simulink model "QuadCentreClosedCoupling"  (R2022b)
settings: Solver=ode4  StartTime=0.0  StopTime=10  FixedStep=1e-3  RelTol=1e-3
undefined symbols (not defined in the file): t1, t2, Vus0
settings Model: Creator=Serious Chimp  LastModifiedBy=Serious Chimp
settings SolverCC: EnableFixedStepZeroCrossing=on
settings OptimizationCC: ReuseModelBlockBuffer=on

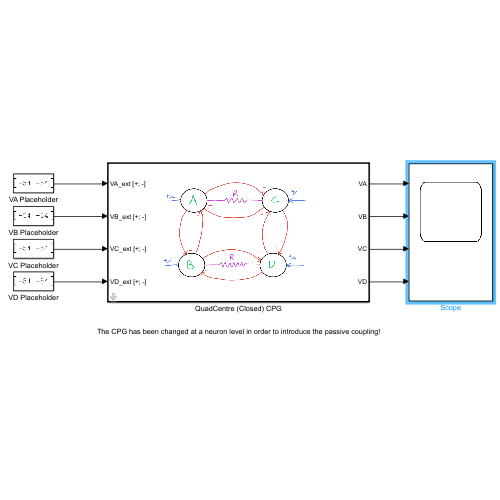
[thumbnail: Simulink's stored preview of the top-level diagram]
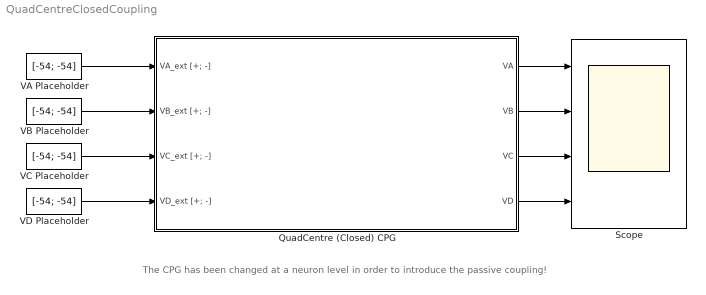
== system QuadCentreClosedCoupling ==
  note: The CPG has been changed at a neuron level in order to introduce the passive coupling!
  QuadCentre (Closed) CPG : Subsystem  TreatAsAtomicUnit=on  mask{tau_s_A=t1, tau_us_A=t2, gSyn_excitatory_A=0.5, gSyn_inhibitory_A=0.5, tauSyn_excitatory_A=50, tauSyn_inhibitory_A=50, GB_A=-40, tau_s_B=t1, tau_us_B=t2, gSyn_excitatory_B=0.5, gSyn_inhibitory_B=0.5, tauSyn_excitatory_B=50, tauSyn_inhibitory_B=50, GB_B=-35, tau_s_C=t1, tau_us_C=t2, gSyn_excitatory_C=0.5, gSyn_inhibitory_C=0.5, tauSyn_excitatory_C=50, tauSyn_inhibitory_C=50, GB_C=-35, tau_s_D=t1, tau_us_D=t2, gSyn_excitatory_D=0.5, gSyn_inhibitory_D=0.5, tauSyn_excitatory_D=50, tauSyn_inhibitory_D=50, GB_D=-40, GB_excitatory=-40, R=200}
      mask prompts: tau_s_A "A - tau_s"; tau_us_A "A - tau_us"; gSyn_excitatory_A "A - Excitatory Synaptic Conductance, gSyn_excitatory"; gSyn_inhibitory_A "A - Inhibitory Synaptic Conductance, gSyn_inhibitory"; tauSyn_excitatory_A "A - Excitatory Synaptic Time Constant, tauSyn_excitatory"; tauSyn_inhibitory_A "A - Inhibitory Synaptic Time Constant, tauSyn_inhibitory"; GB_A "A - Inhibitory Synapse Threshold, GB_A"; tau_s_B "B - tau_s"; tau_us_B "B - tau_us"; gSyn_excitatory_B "B - Excitatory Synaptic Conductance, gSyn_excitatory"; gSyn_inhibitory_B "B - Inhibitory Synaptic Conductance, gSyn_inhibitory"; tauSyn_excitatory_B "B - Excitatory Synaptic Time Constant, tauSyn_excitatory"; tauSyn_inhibitory_B "B - Inhibitory Synaptic Time Constant, tauSyn_inhibitory"; GB_B "B - Inhibitory Synapse Threshold, GB_B"; tau_s_C "C - tau_s"; tau_us_C "C - tau_us"; gSyn_excitatory_C "C - Excitatory Synaptic Conductance, gSyn_excitatory"; gSyn_inhibitory_C "C - Inhibitory Synaptic Conductance, gSyn_inhibitory"; tauSyn_excitatory_C "C - Excitatory Synaptic Time Constant, tauSyn_excitatory"; tauSyn_inhibitory_C "C - Inhibitory Synaptic Time Constant, tauSyn_inhibitory"; GB_C "C - Inhibitory Synapse Threshold, GB_C"; tau_s_D "D - tau_s"; tau_us_D "D - tau_us"; gSyn_excitatory_D "D - Excitatory Synaptic Conductance, gSyn_excitatory"; gSyn_inhibitory_D "D - Inhibitory Synaptic Conductance, gSyn_inhibitory"; tauSyn_excitatory_D "D - Excitatory Synaptic Time Constant, tauSyn_excitatory"; tauSyn_inhibitory_D "D - Inhibitory Synaptic Time Constant, tauSyn_inhibitory"; GB_D "D - Inhibitory Synapse Threshold, GB_D"; GB_excitatory "Excitatory Synapse Gate Threshold, GB_excitatory"; R "Coupling Resistance, R"
      mask Display: image('$imagefile'); % Use "Edit Image" on toolstrip to change.
  Scope : Scope  NumInputPorts=4
  VA Placeholder : Constant  Value=[-54; -54]
  VB Placeholder : Constant  Value=[-54; -54]
  VC Placeholder : Constant  Value=[-54; -54]
  VD Placeholder : Constant  Value=[-54; -54]
  wires:
  QuadCentre (Closed) CPG/1(VA) -> Scope/1
  QuadCentre (Closed) CPG/2(VB) -> Scope/2
  QuadCentre (Closed) CPG/3(VC) -> Scope/3
  QuadCentre (Closed) CPG/4(VD) -> Scope/4
  VA Placeholder/1 -> QuadCentre (Closed) CPG/1(VA_ext [+; -])
  VB Placeholder/1 -> QuadCentre (Closed) CPG/2(VB_ext [+; -])
  VD Placeholder/1 -> QuadCentre (Closed) CPG/4(VD_ext [+; -])
  VC Placeholder/1 -> QuadCentre (Closed) CPG/3(VC_ext [+; -])

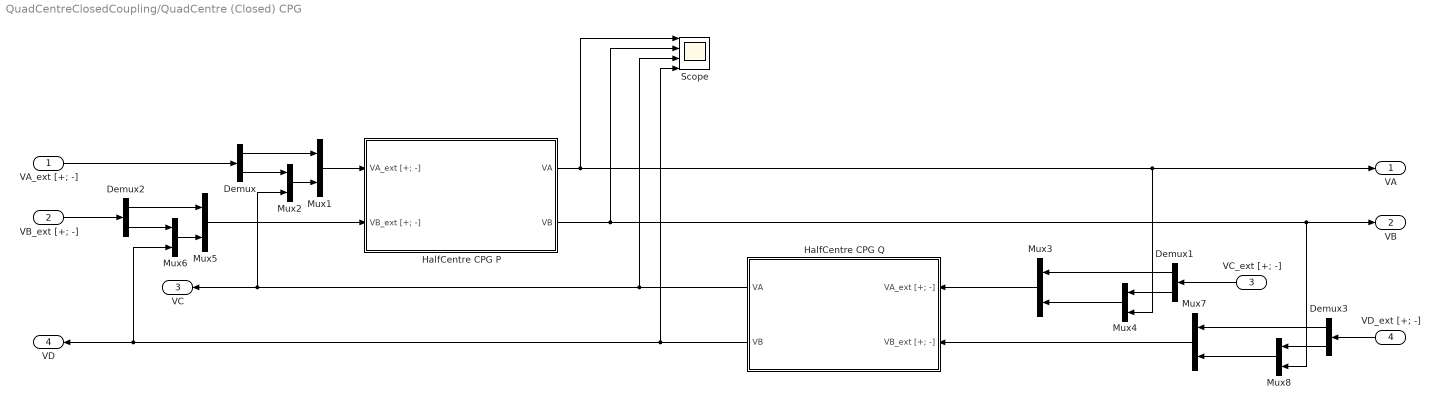
== system QuadCentreClosedCoupling/QuadCentre (Closed) CPG ==
  VA_ext [+; -] : Inport
  VB_ext [+; -] : Inport  Port=2
  VC_ext [+; -] : Inport  Port=3
  VD_ext [+; -] : Inport  Port=4
  Demux{,1..3} (4 alike) : Demux  Outputs=2
  HalfCentre CPG P : Subsystem  TreatAsAtomicUnit=on  mask{tau_s_A=t1, tau_us_A=t2, gSyn_excitatory_A=gSyn_excitatory_A, gSyn_inhibitory_A=gSyn_inhibitory_A, tauSyn_excitatory_A=tauSyn_excitatory_A, tauSyn_inhibitory_A=tauSyn_inhibitory_A, GB_A=GB_A, tau_s_B=t1, tau_us_B=t2, gSyn_excitatory_B=gSyn_excitatory_B, gSyn_inhibitory_B=gSyn_inhibitory_B, tauSyn_excitatory_B=tauSyn_excitatory_B, tauSyn_inhibitory_B=tauSyn_inhibitory_B, GB_B=GB_B, GB_excitatory=GB_excitatory}
      mask prompts: tau_s_A "A - tau_s"; tau_us_A "A - tau_us"; gSyn_excitatory_A "A - Excitatory Synaptic Conductance, gSyn_excitatory"; gSyn_inhibitory_A "A - Inhibitory Synaptic Conductance, gSyn_inhibitory"; tauSyn_excitatory_A "A - Excitatory Synaptic Time Constant, tauSyn_excitatory"; tauSyn_inhibitory_A "A - Inhibitory Synaptic Time Constant, tauSyn_inhibitory"; GB_A "A - Inhibitory Synapse Threshold, GB_A"; tau_s_B "B - tau_s"; tau_us_B "B - tau_us"; gSyn_excitatory_B "B - Excitatory Synaptic Conductance, gSyn_excitatory"; gSyn_inhibitory_B "B - Inhibitory Synaptic Conductance, gSyn_inhibitory"; tauSyn_excitatory_B "B - Excitatory Synaptic Time Constant, tauSyn_excitatory"; tauSyn_inhibitory_B "B - Inhibitory Synaptic Time Constant, tauSyn_inhibitory"; GB_B "B - Inhibitory Synapse Threshold, GB_B"; GB_excitatory "Excitatory Gate Biases, GB_excitatory"
      mask Display: image('$imagefile'); % Use "Edit Image" on toolstrip to change.
  HalfCentre CPG Q : Subsystem  TreatAsAtomicUnit=on  mask{tau_s_A=t1, tau_us_A=t2, gSyn_excitatory_A=gSyn_excitatory_C, gSyn_inhibitory_A=gSyn_inhibitory_C, tauSyn_excitatory_A=tauSyn_excitatory_C, tauSyn_inhibitory_A=tauSyn_inhibitory_C, GB_A=GB_C, tau_s_B=t1, tau_us_B=t2, gSyn_excitatory_B=gSyn_excitatory_D, gSyn_inhibitory_B=gSyn_inhibitory_D, tauSyn_excitatory_B=tauSyn_excitatory_D, tauSyn_inhibitory_B=tauSyn_inhibitory_D, GB_B=GB_D, GB_excitatory=GB_excitatory}
      mask prompts: tau_s_A "A - tau_s"; tau_us_A "A - tau_us"; gSyn_excitatory_A "A - Excitatory Synaptic Conductance, gSyn_excitatory"; gSyn_inhibitory_A "A - Inhibitory Synaptic Conductance, gSyn_inhibitory"; tauSyn_excitatory_A "A - Excitatory Synaptic Time Constant, tauSyn_excitatory"; tauSyn_inhibitory_A "A - Inhibitory Synaptic Time Constant, tauSyn_inhibitory"; GB_A "A - Inhibitory Synapse Threshold, GB_A"; tau_s_B "B - tau_s"; tau_us_B "B - tau_us"; gSyn_excitatory_B "B - Excitatory Synaptic Conductance, gSyn_excitatory"; gSyn_inhibitory_B "B - Inhibitory Synaptic Conductance, gSyn_inhibitory"; tauSyn_excitatory_B "B - Excitatory Synaptic Time Constant, tauSyn_excitatory"; tauSyn_inhibitory_B "B - Inhibitory Synaptic Time Constant, tauSyn_inhibitory"; GB_B "B - Inhibitory Synapse Threshold, GB_B"; GB_excitatory "Excitatory Gate Biases, GB_excitatory"
      mask Display: image('$imagefile'); % Use "Edit Image" on toolstrip to change.
  Mux{1..8} (8 alike) : Mux  Inputs=2
  Scope : Scope  NumInputPorts=4
  VA : Outport
  VB : Outport  Port=2
  VC : Outport  Port=3
  VD : Outport  Port=4
  wires:
  Demux3/2 -> Mux8/1
  HalfCentre CPG P/2(VB) -> Mux8/2, VB/1, Scope/2
  Demux1/2 -> Mux4/1
  Demux3/1 -> Mux7/1
  Mux8/1 -> Mux7/2
  VD_ext [+; -]/1 -> Demux3/1
  Mux1/1 -> HalfCentre CPG P/1(VA_ext [+; -])
  Mux3/1 -> HalfCentre CPG Q/1(VA_ext [+; -])
  Demux/1 -> Mux1/1
  Demux2/1 -> Mux5/1
  Demux2/2 -> Mux6/1
  VC_ext [+; -]/1 -> Demux1/1
  Mux2/1 -> Mux1/2
  VB_ext [+; -]/1 -> Demux2/1
  Mux6/1 -> Mux5/2
  VA_ext [+; -]/1 -> Demux/1
  HalfCentre CPG P/1(VA) -> Scope/1, Mux4/2, VA/1
  Demux/2 -> Mux2/1
  Mux7/1 -> HalfCentre CPG Q/2(VB_ext [+; -])
  Mux5/1 -> HalfCentre CPG P/2(VB_ext [+; -])
  Mux4/1 -> Mux3/2
  Demux1/1 -> Mux3/1
  HalfCentre CPG Q/1(VA) -> Scope/3, Mux2/2, VC/1
  HalfCentre CPG Q/2(VB) -> Mux6/2, VD/1, Scope/4

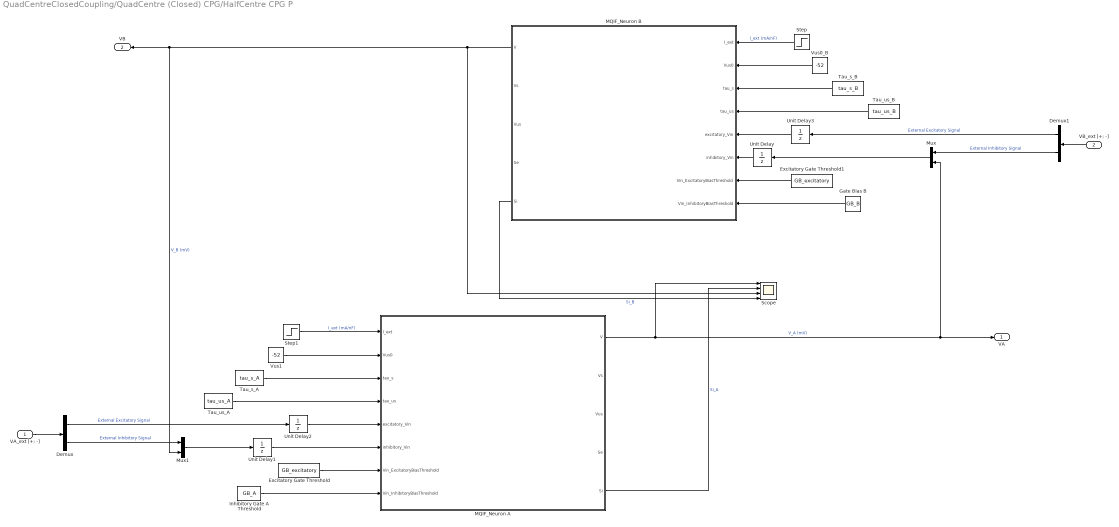
== system QuadCentreClosedCoupling/QuadCentre (Closed) CPG/HalfCentre CPG P ==
  VA_ext [+; -] : Inport
  VB_ext [+; -] : Inport  Port=2
  Demux : Demux  Outputs=2
  Demux1 : Demux  Outputs=2
  Excitatory Gate Threshold : Constant  Value=GB_excitatory
  Excitatory Gate Threshold1 : Constant  Value=GB_excitatory
  Gate BIas B : Constant  Value=GB_B
  Inhibitory Gate A Threshold : Constant  Value=GB_A
  MQIF_Neuron A : Subsystem  TreatAsAtomicUnit=on  mask{V0=-52, Vs0=-50, V_threshold=20, V_reset=-45, Vs_reset=7.5, delta_Vus=1.7, g_f=1.0, g_s=0.5, g_us=0.015, C=0.82, Ve_syn=0, Vi_syn=-90, g_syn_excitatory=gSyn_excitatory_A, g_syn_inhibitory=gSyn_inhibitory_A, tauSyn_excitatory=tauSyn_excitatory_A, tauSyn_inhibitory=tauSyn_inhibitory_A, k=250}
      mask prompts: V0 "Equilibrium V0"; Vs0 "Equilibrium Vs0"; V_threshold "Threshold for Spike, V_thresh"; V_reset "After-spike Reset Votlage, V_r"; Vs_reset "After-spike Reset Vs, Vs_r"; delta_Vus "Vus After-spike Memory, delta_Vus"; g_f "I Conductance, g_f"; g_s "I_us Conductance, g_s"; g_us "I_us Conductance, g_us"; C "Capacitance, C"; Ve_syn "Equilibrium Inhibitory Synapse Voltage, Ve_syn"; Vi_syn "Equilibrium Inhibitory Synapse Voltage, Vi_syn"; g_syn_excitatory "Excitatory Synapse Conductance, g_syn_excitatory"; g_syn_inhibitory "Inhibitory Synapse Conductance, g_syn_inhibitory"; tauSyn_excitatory "Excitatory Synapse Time Constant, tauSyn_excitatory"; tauSyn_inhibitory "Inhibitory Synapse Time Constant, tauSyn_inhibitory"; k "Speed/Rate Constant, k"
      mask DialogControl NeuronStateVariables Prompt: Parameters
  MQIF_Neuron B : Subsystem  TreatAsAtomicUnit=on  mask{V0=-52, Vs0=-50, V_threshold=20, V_reset=-45, Vs_reset=7.5, delta_Vus=1.7, g_f=1.0, g_s=0.5, g_us=0.015, C=0.82, Ve_syn=0, Vi_syn=-90, g_syn_excitatory=gSyn_excitatory_B, g_syn_inhibitory=gSyn_inhibitory_B, tauSyn_excitatory=tauSyn_excitatory_B, tauSyn_inhibitory=tauSyn_inhibitory_B, k=250}
      mask prompts: V0 "Equilibrium V0"; Vs0 "Equilibrium Vs0"; V_threshold "Threshold for Spike, V_thresh"; V_reset "After-spike Reset Votlage, V_r"; Vs_reset "After-spike Reset Vs, Vs_r"; delta_Vus "Vus After-spike Memory, delta_Vus"; g_f "I Conductance, g_f"; g_s "I_us Conductance, g_s"; g_us "I_us Conductance, g_us"; C "Capacitance, C"; Ve_syn "Equilibrium Inhibitory Synapse Voltage, Ve_syn"; Vi_syn "Equilibrium Inhibitory Synapse Voltage, Vi_syn"; g_syn_excitatory "Excitatory Synapse Conductance, g_syn_excitatory"; g_syn_inhibitory "Inhibitory Synapse Conductance, g_syn_inhibitory"; tauSyn_excitatory "Excitatory Synapse Time Constant, tauSyn_excitatory"; tauSyn_inhibitory "Inhibitory Synapse Time Constant, tauSyn_inhibitory"; k "Speed/Rate Constant, k"
      mask DialogControl NeuronStateVariables Prompt: Parameters
  Mux : Mux  Inputs=2
  Mux1 : Mux  Inputs=2
  Scope : Scope  NumInputPorts=4
  Step : Step  After=5  SampleTime=0
  Step1 : Step  After=5  SampleTime=0
  Tau_s_A : Constant  Value=tau_s_A
  Tau_s_B : Constant  Value=tau_s_B
  Tau_us_A : Constant  Value=tau_us_A
  Tau_us_B : Constant  Value=tau_us_B
  Unit Delay : UnitDelay  InitialCondition=[-54; -54]  SampleTime=-1  HasFrameUpgradeWarning=on
  Unit Delay1 : UnitDelay  InitialCondition=[-54; -54]  SampleTime=-1  HasFrameUpgradeWarning=on
  Unit Delay2 : UnitDelay  InitialCondition=-54  SampleTime=-1  HasFrameUpgradeWarning=on
  Unit Delay3 : UnitDelay  InitialCondition=-54  SampleTime=-1  HasFrameUpgradeWarning=on
  Vus0_B : Constant  Value=-52
  Vus1 : Constant  Value=-52
  VA : Outport
  VB : Outport  Port=2
  wires:
  Vus0_B/1 -> MQIF_Neuron B/2(Vus0)
  Unit Delay/1 -> MQIF_Neuron B/6(inhibitory_Vin)
  Inhibitory Gate A Threshold/1 -> MQIF_Neuron A/8(Vin_InhibitoryBiasThreshold)
  Tau_us_B/1 -> MQIF_Neuron B/4(tau_us)
  Vus1/1 -> MQIF_Neuron A/2(Vus0)
  Step1/1 -> MQIF_Neuron A/1(I_ext)  "I_ext (mA/nF)"
  Tau_s_A/1 -> MQIF_Neuron A/3(tau_s)
  Tau_s_B/1 -> MQIF_Neuron B/3(tau_s)
  Tau_us_A/1 -> MQIF_Neuron A/4(tau_us)
  Step/1 -> MQIF_Neuron B/1(I_ext)  "I_ext (mA/nF)"
  Unit Delay1/1 -> MQIF_Neuron A/6(inhibitory_Vin)
  Gate BIas B/1 -> MQIF_Neuron B/8(Vin_InhibitoryBiasThreshold)
  VB_ext [+; -]/1 -> Demux1/1
  Mux/1 -> Unit Delay/1
  Mux1/1 -> Unit Delay1/1
  VA_ext [+; -]/1 -> Demux/1
  Excitatory Gate Threshold/1 -> MQIF_Neuron A/7(Vin_ExcitatoryBiasThreshold)
  Demux/1 -> Unit Delay2/1  "External Excitatory Signal"
  MQIF_Neuron A/1(V) -> Scope/1, VA/1, Mux/2  "V_A (mV)"
  Unit Delay3/1 -> MQIF_Neuron B/5(excitatory_Vin)
  Demux/2 -> Mux1/1  "External Inhibitory Signal"
  Unit Delay2/1 -> MQIF_Neuron A/5(excitatory_Vin)
  Demux1/2 -> Mux/1  "External Inhibitory Signal"
  Demux1/1 -> Unit Delay3/1  "External Excitatory Signal"
  Excitatory Gate Threshold1/1 -> MQIF_Neuron B/7(Vin_ExcitatoryBiasThreshold)
  MQIF_Neuron B/1(V) -> Scope/3, VB/1, Mux1/2  "V_B (mV)"
  MQIF_Neuron A/5(Si) -> Scope/2  "Si_A"
  MQIF_Neuron B/5(Si) -> Scope/4  "Si_B"

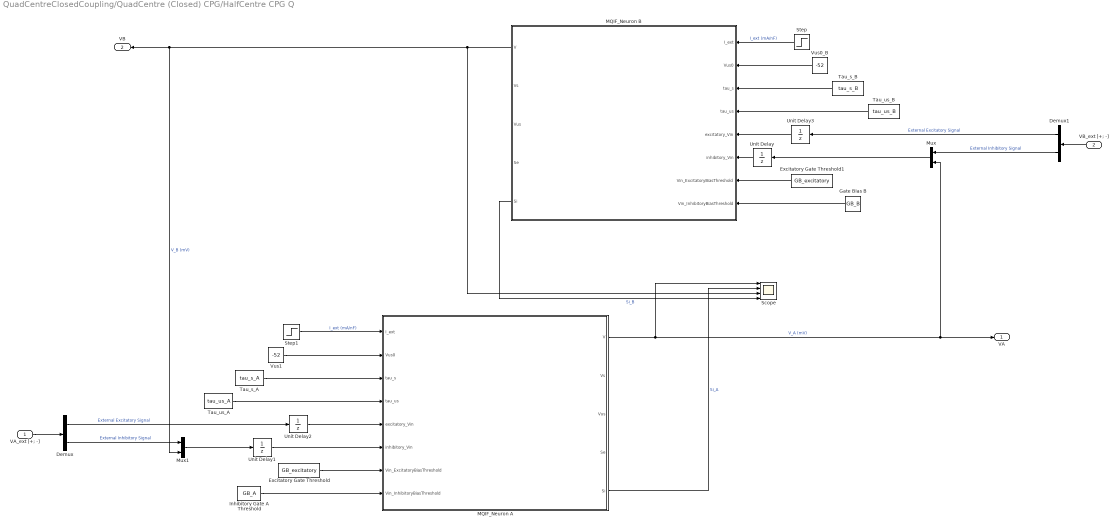
== system QuadCentreClosedCoupling/QuadCentre (Closed) CPG/HalfCentre CPG Q ==
  VA_ext [+; -] : Inport
  VB_ext [+; -] : Inport  Port=2
  Demux : Demux  Outputs=2
  Demux1 : Demux  Outputs=2
  Excitatory Gate Threshold : Constant  Value=GB_excitatory
  Excitatory Gate Threshold1 : Constant  Value=GB_excitatory
  Gate BIas B : Constant  Value=GB_B
  Inhibitory Gate A Threshold : Constant  Value=GB_A
  MQIF_Neuron A : Subsystem  TreatAsAtomicUnit=on  mask{V0=-52, Vs0=-50, V_threshold=20, V_reset=-45, Vs_reset=7.5, delta_Vus=1.7, g_f=1.0, g_s=0.5, g_us=0.015, C=0.82, Ve_syn=0, Vi_syn=-90, g_syn_excitatory=gSyn_excitatory_C, g_syn_inhibitory=gSyn_inhibitory_C, tauSyn_excitatory=tauSyn_excitatory_C, tauSyn_inhibitory=tauSyn_inhibitory_C, k=250}
      mask prompts: V0 "Equilibrium V0"; Vs0 "Equilibrium Vs0"; V_threshold "Threshold for Spike, V_thresh"; V_reset "After-spike Reset Votlage, V_r"; Vs_reset "After-spike Reset Vs, Vs_r"; delta_Vus "Vus After-spike Memory, delta_Vus"; g_f "I Conductance, g_f"; g_s "I_us Conductance, g_s"; g_us "I_us Conductance, g_us"; C "Capacitance, C"; Ve_syn "Equilibrium Inhibitory Synapse Voltage, Ve_syn"; Vi_syn "Equilibrium Inhibitory Synapse Voltage, Vi_syn"; g_syn_excitatory "Excitatory Synapse Conductance, g_syn_excitatory"; g_syn_inhibitory "Inhibitory Synapse Conductance, g_syn_inhibitory"; tauSyn_excitatory "Excitatory Synapse Time Constant, tauSyn_excitatory"; tauSyn_inhibitory "Inhibitory Synapse Time Constant, tauSyn_inhibitory"; k "Speed/Rate Constant, k"
      mask DialogControl NeuronStateVariables Prompt: Parameters
  MQIF_Neuron B : Subsystem  TreatAsAtomicUnit=on  mask{V0=-52, Vs0=-50, V_threshold=20, V_reset=-45, Vs_reset=7.5, delta_Vus=1.7, g_f=1.0, g_s=0.5, g_us=0.015, C=0.82, Ve_syn=0, Vi_syn=-90, g_syn_excitatory=gSyn_excitatory_D, g_syn_inhibitory=gSyn_inhibitory_D, tauSyn_excitatory=tauSyn_excitatory_D, tauSyn_inhibitory=tauSyn_inhibitory_D, k=250}
      mask prompts: V0 "Equilibrium V0"; Vs0 "Equilibrium Vs0"; V_threshold "Threshold for Spike, V_thresh"; V_reset "After-spike Reset Votlage, V_r"; Vs_reset "After-spike Reset Vs, Vs_r"; delta_Vus "Vus After-spike Memory, delta_Vus"; g_f "I Conductance, g_f"; g_s "I_us Conductance, g_s"; g_us "I_us Conductance, g_us"; C "Capacitance, C"; Ve_syn "Equilibrium Inhibitory Synapse Voltage, Ve_syn"; Vi_syn "Equilibrium Inhibitory Synapse Voltage, Vi_syn"; g_syn_excitatory "Excitatory Synapse Conductance, g_syn_excitatory"; g_syn_inhibitory "Inhibitory Synapse Conductance, g_syn_inhibitory"; tauSyn_excitatory "Excitatory Synapse Time Constant, tauSyn_excitatory"; tauSyn_inhibitory "Inhibitory Synapse Time Constant, tauSyn_inhibitory"; k "Speed/Rate Constant, k"
      mask DialogControl NeuronStateVariables Prompt: Parameters
  Mux : Mux  Inputs=2
  Mux1 : Mux  Inputs=2
  Scope : Scope  NumInputPorts=4
  Step : Step  After=5  SampleTime=0
  Step1 : Step  After=5  SampleTime=0
  Tau_s_A : Constant  Value=tau_s_A
  Tau_s_B : Constant  Value=tau_s_B
  Tau_us_A : Constant  Value=tau_us_A
  Tau_us_B : Constant  Value=tau_us_B
  Unit Delay : UnitDelay  InitialCondition=[-54; -54]  SampleTime=-1  HasFrameUpgradeWarning=on
  Unit Delay1 : UnitDelay  InitialCondition=[-54; -54]  SampleTime=-1  HasFrameUpgradeWarning=on
  Unit Delay2 : UnitDelay  InitialCondition=-54  SampleTime=-1  HasFrameUpgradeWarning=on
  Unit Delay3 : UnitDelay  InitialCondition=-54  SampleTime=-1  HasFrameUpgradeWarning=on
  Vus0_B : Constant  Value=-52
  Vus1 : Constant  Value=-52
  VA : Outport
  VB : Outport  Port=2
  wires:
  Vus0_B/1 -> MQIF_Neuron B/2(Vus0)
  Unit Delay/1 -> MQIF_Neuron B/6(inhibitory_Vin)
  Inhibitory Gate A Threshold/1 -> MQIF_Neuron A/8(Vin_InhibitoryBiasThreshold)
  Tau_us_B/1 -> MQIF_Neuron B/4(tau_us)
  Vus1/1 -> MQIF_Neuron A/2(Vus0)
  Step1/1 -> MQIF_Neuron A/1(I_ext)  "I_ext (mA/nF)"
  Tau_s_A/1 -> MQIF_Neuron A/3(tau_s)
  Tau_s_B/1 -> MQIF_Neuron B/3(tau_s)
  Tau_us_A/1 -> MQIF_Neuron A/4(tau_us)
  Step/1 -> MQIF_Neuron B/1(I_ext)  "I_ext (mA/nF)"
  Unit Delay1/1 -> MQIF_Neuron A/6(inhibitory_Vin)
  Gate BIas B/1 -> MQIF_Neuron B/8(Vin_InhibitoryBiasThreshold)
  VB_ext [+; -]/1 -> Demux1/1
  Mux/1 -> Unit Delay/1
  Mux1/1 -> Unit Delay1/1
  VA_ext [+; -]/1 -> Demux/1
  Excitatory Gate Threshold/1 -> MQIF_Neuron A/7(Vin_ExcitatoryBiasThreshold)
  Demux/1 -> Unit Delay2/1  "External Excitatory Signal"
  MQIF_Neuron A/1(V) -> Scope/1, VA/1, Mux/2  "V_A (mV)"
  Unit Delay3/1 -> MQIF_Neuron B/5(excitatory_Vin)
  Demux/2 -> Mux1/1  "External Inhibitory Signal"
  Unit Delay2/1 -> MQIF_Neuron A/5(excitatory_Vin)
  Demux1/2 -> Mux/1  "External Inhibitory Signal"
  Demux1/1 -> Unit Delay3/1  "External Excitatory Signal"
  Excitatory Gate Threshold1/1 -> MQIF_Neuron B/7(Vin_ExcitatoryBiasThreshold)
  MQIF_Neuron B/1(V) -> Scope/3, VB/1, Mux1/2  "V_B (mV)"
  MQIF_Neuron A/5(Si) -> Scope/2  "Si_A"
  MQIF_Neuron B/5(Si) -> Scope/4  "Si_B"

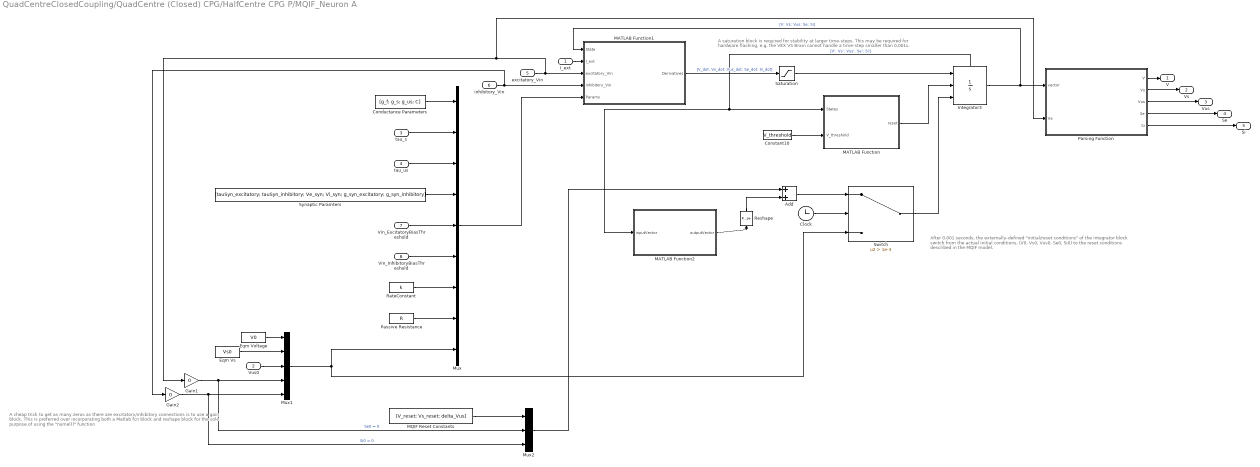
== system QuadCentreClosedCoupling/QuadCentre (Closed) CPG/HalfCentre CPG P/MQIF_Neuron A ==
  note: A saturation block is required for stability at larger time-steps. This may be required for hardware flashing, e.g. the VEX V5 Brain cannot handle a time-step smaller than 0.001s.
  note: After 0.001 seconds, the externally-defined "initial/reset conditions" of the integrator block switch from the actual initial conditions, (V0, Vs0, Vus0, Se0, Si0) to the reset conditions described in the MQIF model.
  note: A cheap trick to get as many zeros as there are excitatory/inhibitory connections
      | is to use a gain block. This is preferred over incorporating both a Matlab fcn block and reshape block for the sole purpose of using the "numel()" function
  I_ext : Inport
  Vus0 : Inport  Port=2
  tau_s : Inport  Port=3
  tau_us : Inport  Port=4
  excitatory_Vin : Inport  Port=5
  inhibitory_Vin : Inport  Port=6
  Vin_ExcitatoryBiasThreshold : Inport  Port=7
  Vin_InhibitoryBiasThreshold : Inport  Port=8
  Add : Sum
  Clock : Clock
  Conductance Parameters : Constant  Value=[g_f; g_s; g_us; C]
  Constant10 : Constant  Value=V_threshold
  Eqm Voltage : Constant  Value=V0
  Eqm Vs : Constant  Value=Vs0
  Gain1 : Gain  Gain=0
  Gain2 : Gain  Gain=0
  Integrator3 : Integrator  ExternalReset=rising  InitialConditionSource=external  InitialCondition=[V0 Vs0 Vus0]  ShowStatePort=on
  MATLAB Function : MATLAB Function  TreatAsAtomicUnit=on
  MATLAB Function1 : MATLAB Function  TreatAsAtomicUnit=on
  MATLAB Function2 : MATLAB Function  TreatAsAtomicUnit=on
  MQIF Reset Constants : Constant  Value=[V_reset; Vs_reset; delta_Vus]
  Mux : Mux  Inputs=9
  Mux1 : Mux  Inputs=5
  Mux2 : Mux  Inputs=3
  Parsing Function : MATLAB Function  TreatAsAtomicUnit=on
  Passive Resistance : Constant  Value=R
  RateConstant : Constant  Value=k
  Reshape : Reshape
  Saturation : Saturate  UpperLimit=1e4  LowerLimit=-1e4  LinearizeAsGain=off  ZeroCross=off
  Switch : Switch  Criteria=u2 > Threshold  Threshold=1e-3  SaturateOnIntegerOverflow=off  InputSameDT=off
  Synaptic Paramters : Constant  Value=[tauSyn_excitatory; tauSyn_inhibitory; Ve_syn; Vi_syn; g_syn_excitatory; g_syn_inhibitory]
  V : Outport
  Vs : Outport  Port=2
  Vus : Outport  Port=3
  Se : Outport  Port=4
  Si : Outport  Port=5
  wires:
  I_ext/1 -> MATLAB Function1/2(I_ext)
  Eqm Voltage/1 -> Mux1/1
  Vus0/1 -> Mux1/3
  Conductance Parameters/1 -> Mux/1
  tau_s/1 -> Mux/2
  tau_us/1 -> Mux/3
  Synaptic Paramters/1 -> Mux/4
  Mux/1 -> MATLAB Function1/5(Params)
  Constant10/1 -> MATLAB Function/2(V_threshold)
  Integrator3/1 -> MATLAB Function1/1(State), Parsing Function/1(vector)  "[V; Vs; Vus; Se; Si]"
  MATLAB Function/1(reset) -> Integrator3/2
  Clock/1 -> Switch/2
  MQIF Reset Constants/1 -> Mux2/1
  Switch/1 -> Integrator3/3
  MATLAB Function2/1(outputVector) -> Reshape/1
  MATLAB Function1/1(Derivatives) -> Saturation/1  "[V_dot; Vs_dot; Vus_dot; Se_dot; Si_dot]"
  Add/1 -> Switch/1
  Eqm Vs/1 -> Mux1/2
  inhibitory_Vin/1 -> Gain2/1, MATLAB Function1/4(inhibitory_Vin)
  Integrator3/State -> MATLAB Function2/1(inputVector), MATLAB Function/1(States)  "[V'; Vs'; Vus'; Se'; Si']"
  Vin_ExcitatoryBiasThreshold/1 -> Mux/5
  Saturation/1 -> Integrator3/1
  excitatory_Vin/1 -> Parsing Function/2(Ve), Gain1/1, MATLAB Function1/3(excitatory_Vin)
  RateConstant/1 -> Mux/7
  Mux1/1 -> Mux/9, Switch/3
  Vin_InhibitoryBiasThreshold/1 -> Mux/6
  Gain1/1 -> Mux1/4, Mux2/2  "Se0 = 0"
  Gain2/1 -> Mux2/3, Mux1/5  "Si0 = 0"
  Mux2/1 -> Add/1
  Reshape/1 -> Add/2
  Parsing Function/3(Vus) -> Vus/1
  Parsing Function/2(Vs) -> Vs/1
  Parsing Function/1(V) -> V/1
  Parsing Function/5(Si) -> Si/1
  Parsing Function/4(Se) -> Se/1
  Passive Resistance/1 -> Mux/8

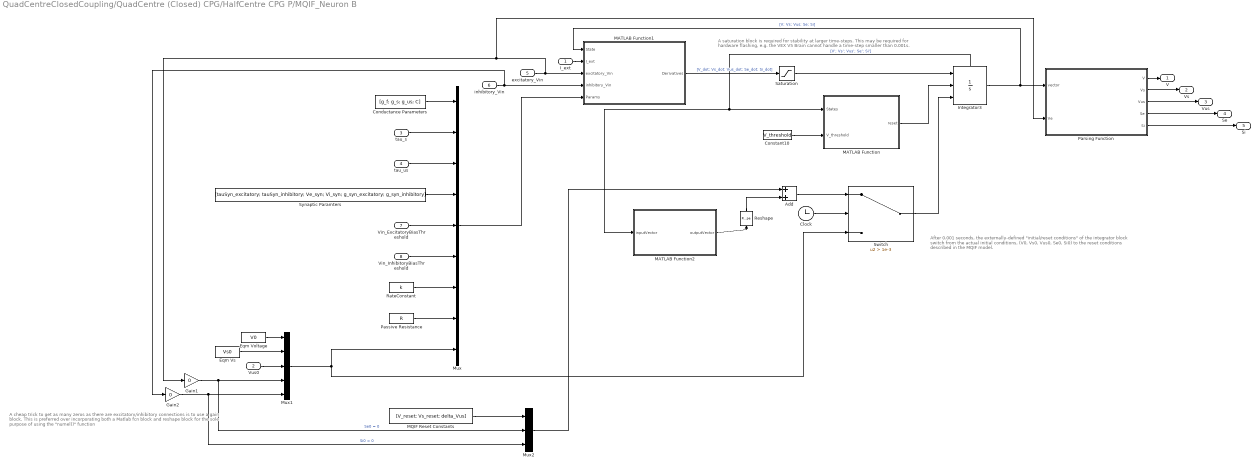
== system QuadCentreClosedCoupling/QuadCentre (Closed) CPG/HalfCentre CPG P/MQIF_Neuron B ==
  note: A saturation block is required for stability at larger time-steps. This may be required for hardware flashing, e.g. the VEX V5 Brain cannot handle a time-step smaller than 0.001s.
  note: After 0.001 seconds, the externally-defined "initial/reset conditions" of the integrator block switch from the actual initial conditions, (V0, Vs0, Vus0, Se0, Si0) to the reset conditions described in the MQIF model.
  note: A cheap trick to get as many zeros as there are excitatory/inhibitory connections
      | is to use a gain block. This is preferred over incorporating both a Matlab fcn block and reshape block for the sole purpose of using the "numel()" function
  I_ext : Inport
  Vus0 : Inport  Port=2
  tau_s : Inport  Port=3
  tau_us : Inport  Port=4
  excitatory_Vin : Inport  Port=5
  inhibitory_Vin : Inport  Port=6
  Vin_ExcitatoryBiasThreshold : Inport  Port=7
  Vin_InhibitoryBiasThreshold : Inport  Port=8
  Add : Sum
  Clock : Clock
  Conductance Parameters : Constant  Value=[g_f; g_s; g_us; C]
  Constant10 : Constant  Value=V_threshold
  Eqm Voltage : Constant  Value=V0
  Eqm Vs : Constant  Value=Vs0
  Gain1 : Gain  Gain=0
  Gain2 : Gain  Gain=0
  Integrator3 : Integrator  ExternalReset=rising  InitialConditionSource=external  InitialCondition=[V0 Vs0 Vus0]  ShowStatePort=on
  MATLAB Function : MATLAB Function  TreatAsAtomicUnit=on
  MATLAB Function1 : MATLAB Function  TreatAsAtomicUnit=on
  MATLAB Function2 : MATLAB Function  TreatAsAtomicUnit=on
  MQIF Reset Constants : Constant  Value=[V_reset; Vs_reset; delta_Vus]
  Mux : Mux  Inputs=9
  Mux1 : Mux  Inputs=5
  Mux2 : Mux  Inputs=3
  Parsing Function : MATLAB Function  TreatAsAtomicUnit=on
  Passive Resistance : Constant  Value=R
  RateConstant : Constant  Value=k
  Reshape : Reshape
  Saturation : Saturate  UpperLimit=1e4  LowerLimit=-1e4  LinearizeAsGain=off  ZeroCross=off
  Switch : Switch  Criteria=u2 > Threshold  Threshold=1e-3  SaturateOnIntegerOverflow=off  InputSameDT=off
  Synaptic Paramters : Constant  Value=[tauSyn_excitatory; tauSyn_inhibitory; Ve_syn; Vi_syn; g_syn_excitatory; g_syn_inhibitory]
  V : Outport
  Vs : Outport  Port=2
  Vus : Outport  Port=3
  Se : Outport  Port=4
  Si : Outport  Port=5
  wires:
  I_ext/1 -> MATLAB Function1/2(I_ext)
  Eqm Voltage/1 -> Mux1/1
  Vus0/1 -> Mux1/3
  Conductance Parameters/1 -> Mux/1
  tau_s/1 -> Mux/2
  tau_us/1 -> Mux/3
  Synaptic Paramters/1 -> Mux/4
  Mux/1 -> MATLAB Function1/5(Params)
  Constant10/1 -> MATLAB Function/2(V_threshold)
  Integrator3/1 -> MATLAB Function1/1(State), Parsing Function/1(vector)  "[V; Vs; Vus; Se; Si]"
  MATLAB Function/1(reset) -> Integrator3/2
  Clock/1 -> Switch/2
  MQIF Reset Constants/1 -> Mux2/1
  Switch/1 -> Integrator3/3
  MATLAB Function2/1(outputVector) -> Reshape/1
  MATLAB Function1/1(Derivatives) -> Saturation/1  "[V_dot; Vs_dot; Vus_dot; Se_dot; Si_dot]"
  Add/1 -> Switch/1
  Eqm Vs/1 -> Mux1/2
  inhibitory_Vin/1 -> Gain2/1, MATLAB Function1/4(inhibitory_Vin)
  Integrator3/State -> MATLAB Function2/1(inputVector), MATLAB Function/1(States)  "[V'; Vs'; Vus'; Se'; Si']"
  Vin_ExcitatoryBiasThreshold/1 -> Mux/5
  Saturation/1 -> Integrator3/1
  excitatory_Vin/1 -> Parsing Function/2(Ve), Gain1/1, MATLAB Function1/3(excitatory_Vin)
  RateConstant/1 -> Mux/7
  Mux1/1 -> Mux/9, Switch/3
  Vin_InhibitoryBiasThreshold/1 -> Mux/6
  Gain1/1 -> Mux1/4, Mux2/2  "Se0 = 0"
  Gain2/1 -> Mux2/3, Mux1/5  "Si0 = 0"
  Mux2/1 -> Add/1
  Reshape/1 -> Add/2
  Parsing Function/3(Vus) -> Vus/1
  Parsing Function/2(Vs) -> Vs/1
  Parsing Function/1(V) -> V/1
  Parsing Function/5(Si) -> Si/1
  Parsing Function/4(Se) -> Se/1
  Passive Resistance/1 -> Mux/8

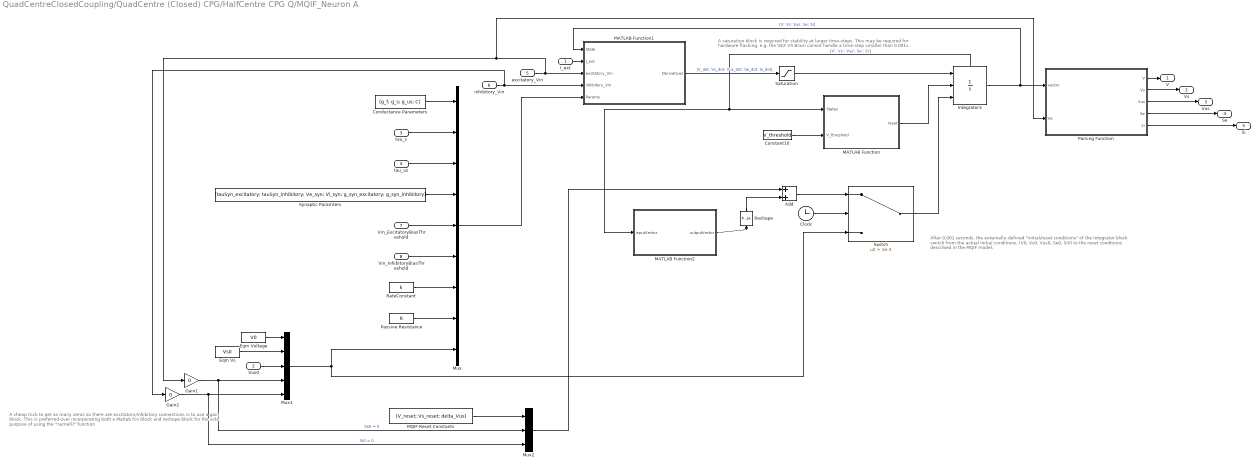
== system QuadCentreClosedCoupling/QuadCentre (Closed) CPG/HalfCentre CPG Q/MQIF_Neuron A ==
  note: A saturation block is required for stability at larger time-steps. This may be required for hardware flashing, e.g. the VEX V5 Brain cannot handle a time-step smaller than 0.001s.
  note: After 0.001 seconds, the externally-defined "initial/reset conditions" of the integrator block switch from the actual initial conditions, (V0, Vs0, Vus0, Se0, Si0) to the reset conditions described in the MQIF model.
  note: A cheap trick to get as many zeros as there are excitatory/inhibitory connections
      | is to use a gain block. This is preferred over incorporating both a Matlab fcn block and reshape block for the sole purpose of using the "numel()" function
  I_ext : Inport
  Vus0 : Inport  Port=2
  tau_s : Inport  Port=3
  tau_us : Inport  Port=4
  excitatory_Vin : Inport  Port=5
  inhibitory_Vin : Inport  Port=6
  Vin_ExcitatoryBiasThreshold : Inport  Port=7
  Vin_InhibitoryBiasThreshold : Inport  Port=8
  Add : Sum
  Clock : Clock
  Conductance Parameters : Constant  Value=[g_f; g_s; g_us; C]
  Constant10 : Constant  Value=V_threshold
  Eqm Voltage : Constant  Value=V0
  Eqm Vs : Constant  Value=Vs0
  Gain1 : Gain  Gain=0
  Gain2 : Gain  Gain=0
  Integrator3 : Integrator  ExternalReset=rising  InitialConditionSource=external  InitialCondition=[V0 Vs0 Vus0]  ShowStatePort=on
  MATLAB Function : MATLAB Function  TreatAsAtomicUnit=on
  MATLAB Function1 : MATLAB Function  TreatAsAtomicUnit=on
  MATLAB Function2 : MATLAB Function  TreatAsAtomicUnit=on
  MQIF Reset Constants : Constant  Value=[V_reset; Vs_reset; delta_Vus]
  Mux : Mux  Inputs=9
  Mux1 : Mux  Inputs=5
  Mux2 : Mux  Inputs=3
  Parsing Function : MATLAB Function  TreatAsAtomicUnit=on
  Passive Resistance : Constant  Value=R
  RateConstant : Constant  Value=k
  Reshape : Reshape
  Saturation : Saturate  UpperLimit=1e4  LowerLimit=-1e4  LinearizeAsGain=off  ZeroCross=off
  Switch : Switch  Criteria=u2 > Threshold  Threshold=1e-3  SaturateOnIntegerOverflow=off  InputSameDT=off
  Synaptic Paramters : Constant  Value=[tauSyn_excitatory; tauSyn_inhibitory; Ve_syn; Vi_syn; g_syn_excitatory; g_syn_inhibitory]
  V : Outport
  Vs : Outport  Port=2
  Vus : Outport  Port=3
  Se : Outport  Port=4
  Si : Outport  Port=5
  wires:
  I_ext/1 -> MATLAB Function1/2(I_ext)
  Eqm Voltage/1 -> Mux1/1
  Vus0/1 -> Mux1/3
  Conductance Parameters/1 -> Mux/1
  tau_s/1 -> Mux/2
  tau_us/1 -> Mux/3
  Synaptic Paramters/1 -> Mux/4
  Mux/1 -> MATLAB Function1/5(Params)
  Constant10/1 -> MATLAB Function/2(V_threshold)
  Integrator3/1 -> MATLAB Function1/1(State), Parsing Function/1(vector)  "[V; Vs; Vus; Se; Si]"
  MATLAB Function/1(reset) -> Integrator3/2
  Clock/1 -> Switch/2
  MQIF Reset Constants/1 -> Mux2/1
  Switch/1 -> Integrator3/3
  MATLAB Function2/1(outputVector) -> Reshape/1
  MATLAB Function1/1(Derivatives) -> Saturation/1  "[V_dot; Vs_dot; Vus_dot; Se_dot; Si_dot]"
  Add/1 -> Switch/1
  Eqm Vs/1 -> Mux1/2
  inhibitory_Vin/1 -> Gain2/1, MATLAB Function1/4(inhibitory_Vin)
  Integrator3/State -> MATLAB Function2/1(inputVector), MATLAB Function/1(States)  "[V'; Vs'; Vus'; Se'; Si']"
  Vin_ExcitatoryBiasThreshold/1 -> Mux/5
  Saturation/1 -> Integrator3/1
  excitatory_Vin/1 -> Parsing Function/2(Ve), Gain1/1, MATLAB Function1/3(excitatory_Vin)
  RateConstant/1 -> Mux/7
  Mux1/1 -> Mux/9, Switch/3
  Vin_InhibitoryBiasThreshold/1 -> Mux/6
  Gain1/1 -> Mux1/4, Mux2/2  "Se0 = 0"
  Gain2/1 -> Mux2/3, Mux1/5  "Si0 = 0"
  Mux2/1 -> Add/1
  Reshape/1 -> Add/2
  Parsing Function/3(Vus) -> Vus/1
  Parsing Function/2(Vs) -> Vs/1
  Parsing Function/1(V) -> V/1
  Parsing Function/5(Si) -> Si/1
  Parsing Function/4(Se) -> Se/1
  Passive Resistance/1 -> Mux/8

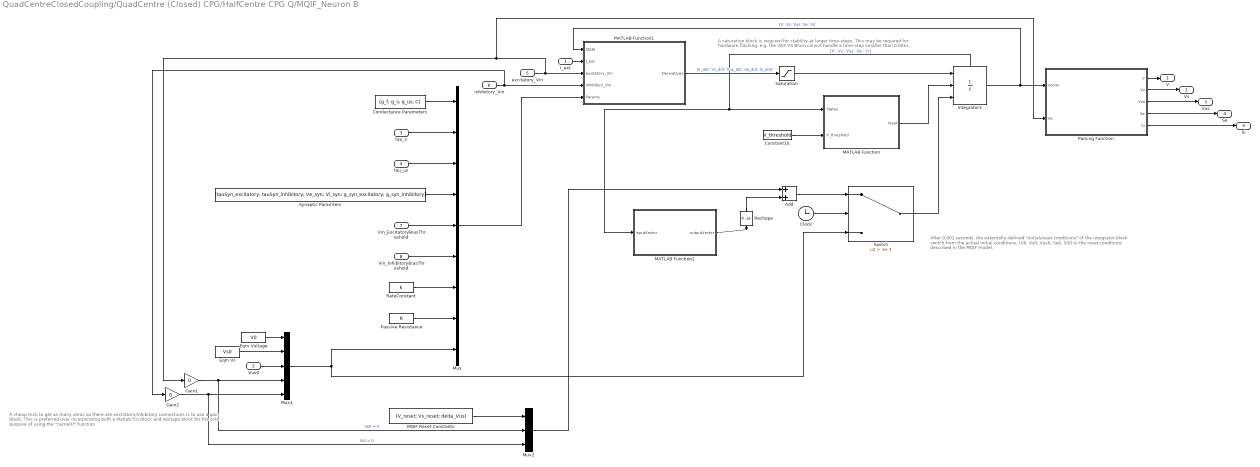
== system QuadCentreClosedCoupling/QuadCentre (Closed) CPG/HalfCentre CPG Q/MQIF_Neuron B ==
  note: A saturation block is required for stability at larger time-steps. This may be required for hardware flashing, e.g. the VEX V5 Brain cannot handle a time-step smaller than 0.001s.
  note: After 0.001 seconds, the externally-defined "initial/reset conditions" of the integrator block switch from the actual initial conditions, (V0, Vs0, Vus0, Se0, Si0) to the reset conditions described in the MQIF model.
  note: A cheap trick to get as many zeros as there are excitatory/inhibitory connections
      | is to use a gain block. This is preferred over incorporating both a Matlab fcn block and reshape block for the sole purpose of using the "numel()" function
  I_ext : Inport
  Vus0 : Inport  Port=2
  tau_s : Inport  Port=3
  tau_us : Inport  Port=4
  excitatory_Vin : Inport  Port=5
  inhibitory_Vin : Inport  Port=6
  Vin_ExcitatoryBiasThreshold : Inport  Port=7
  Vin_InhibitoryBiasThreshold : Inport  Port=8
  Add : Sum
  Clock : Clock
  Conductance Parameters : Constant  Value=[g_f; g_s; g_us; C]
  Constant10 : Constant  Value=V_threshold
  Eqm Voltage : Constant  Value=V0
  Eqm Vs : Constant  Value=Vs0
  Gain1 : Gain  Gain=0
  Gain2 : Gain  Gain=0
  Integrator3 : Integrator  ExternalReset=rising  InitialConditionSource=external  InitialCondition=[V0 Vs0 Vus0]  ShowStatePort=on
  MATLAB Function : MATLAB Function  TreatAsAtomicUnit=on
  MATLAB Function1 : MATLAB Function  TreatAsAtomicUnit=on
  MATLAB Function2 : MATLAB Function  TreatAsAtomicUnit=on
  MQIF Reset Constants : Constant  Value=[V_reset; Vs_reset; delta_Vus]
  Mux : Mux  Inputs=9
  Mux1 : Mux  Inputs=5
  Mux2 : Mux  Inputs=3
  Parsing Function : MATLAB Function  TreatAsAtomicUnit=on
  Passive Resistance : Constant  Value=R
  RateConstant : Constant  Value=k
  Reshape : Reshape
  Saturation : Saturate  UpperLimit=1e4  LowerLimit=-1e4  LinearizeAsGain=off  ZeroCross=off
  Switch : Switch  Criteria=u2 > Threshold  Threshold=1e-3  SaturateOnIntegerOverflow=off  InputSameDT=off
  Synaptic Paramters : Constant  Value=[tauSyn_excitatory; tauSyn_inhibitory; Ve_syn; Vi_syn; g_syn_excitatory; g_syn_inhibitory]
  V : Outport
  Vs : Outport  Port=2
  Vus : Outport  Port=3
  Se : Outport  Port=4
  Si : Outport  Port=5
  wires:
  I_ext/1 -> MATLAB Function1/2(I_ext)
  Eqm Voltage/1 -> Mux1/1
  Vus0/1 -> Mux1/3
  Conductance Parameters/1 -> Mux/1
  tau_s/1 -> Mux/2
  tau_us/1 -> Mux/3
  Synaptic Paramters/1 -> Mux/4
  Mux/1 -> MATLAB Function1/5(Params)
  Constant10/1 -> MATLAB Function/2(V_threshold)
  Integrator3/1 -> MATLAB Function1/1(State), Parsing Function/1(vector)  "[V; Vs; Vus; Se; Si]"
  MATLAB Function/1(reset) -> Integrator3/2
  Clock/1 -> Switch/2
  MQIF Reset Constants/1 -> Mux2/1
  Switch/1 -> Integrator3/3
  MATLAB Function2/1(outputVector) -> Reshape/1
  MATLAB Function1/1(Derivatives) -> Saturation/1  "[V_dot; Vs_dot; Vus_dot; Se_dot; Si_dot]"
  Add/1 -> Switch/1
  Eqm Vs/1 -> Mux1/2
  inhibitory_Vin/1 -> Gain2/1, MATLAB Function1/4(inhibitory_Vin)
  Integrator3/State -> MATLAB Function2/1(inputVector), MATLAB Function/1(States)  "[V'; Vs'; Vus'; Se'; Si']"
  Vin_ExcitatoryBiasThreshold/1 -> Mux/5
  Saturation/1 -> Integrator3/1
  excitatory_Vin/1 -> Parsing Function/2(Ve), Gain1/1, MATLAB Function1/3(excitatory_Vin)
  RateConstant/1 -> Mux/7
  Mux1/1 -> Mux/9, Switch/3
  Vin_InhibitoryBiasThreshold/1 -> Mux/6
  Gain1/1 -> Mux1/4, Mux2/2  "Se0 = 0"
  Gain2/1 -> Mux2/3, Mux1/5  "Si0 = 0"
  Mux2/1 -> Add/1
  Reshape/1 -> Add/2
  Parsing Function/3(Vus) -> Vus/1
  Parsing Function/2(Vs) -> Vs/1
  Parsing Function/1(V) -> V/1
  Parsing Function/5(Si) -> Si/1
  Parsing Function/4(Se) -> Se/1
  Passive Resistance/1 -> Mux/8

== matlab function QuadCentreClosedCoupling/QuadCentre (Closed) CPG/HalfCentre CPG Q/MQIF_Neuron B/MATLAB Function2 ==
  data: inputVector input; outputVector output
% This function is required to make sure that the MQIF neuron is input
% agnostic, (can handle any number of excitatory/inhibitory connections).
% 
% We require a matrix that can extract Vus (scalar), Se and Si (vectors of
% arbitrary length), and ignore the other values. This is because these
% values are "remembered" after each action potential and are required in
% the subsequent resetting of states.

function outputVector = generalisedMatrix(inputVector)
    % Get the size of the input vector
    n = length(inputVector);

    % Create a square matrix of zeros
    Matrix = zeros(n);

    % Set the (3, 3) element to 1
    Matrix(3, 3) = 1;

    % Set the values for every row i, starting from the fourth row
    for i = 4:n
        Matrix(i, i) = 1;
    end

    outputVector = Matrix*inputVector;
end

== matlab function QuadCentreClosedCoupling/QuadCentre (Closed) CPG/HalfCentre CPG Q/MQIF_Neuron B/Parsing Function ==
  data: vector input; V output; Vs output; Vus output; Ve input; Se output; Si output
% This fcn parses through the vectorised input signal, to output the
% various states through the enclosing mask's outports. It is designed to
% be input agnostic, (i.e. the neuron can handle any number of excitatory/inhibitory
% connections, and it outputs Se and Si as vectorised signals).

function [V,Vs,Vus,Se,Si] = InputAgnosticDemux(vector, Ve)
    V = vector(1);
    Vs = vector(2);
    Vus = vector(3);
    Se = vector(4:numel(Ve)+3);
    Si = vector(numel(Ve)+4:end);
end

== matlab function QuadCentreClosedCoupling/QuadCentre (Closed) CPG/HalfCentre CPG P/MQIF_Neuron A/MATLAB Function ==
  data: States input; reset output; V_threshold input
% This fcn triggers the reset of the following integrator block. When membrane
% potential rises above V_threshold, an action potential has been fired, 
% as specified for integrate-and-fire neuron behavior.

function reset = ResetTrigger(States, V_threshold)

V = States(1);

reset = (V > V_threshold);

end

== matlab function QuadCentreClosedCoupling/QuadCentre (Closed) CPG/HalfCentre CPG Q/MQIF_Neuron A/MATLAB Function ==
  data: States input; reset output; V_threshold input
% This fcn triggers the reset of the following integrator block. When membrane
% potential rises above V_threshold, an action potential has been fired, 
% as specified for integrate-and-fire neuron behavior.

function reset = ResetTrigger(States, V_threshold)

V = States(1);

reset = (V > V_threshold);

end

== matlab function QuadCentreClosedCoupling/QuadCentre (Closed) CPG/HalfCentre CPG P/MQIF_Neuron A/MATLAB Function1 ==
  data: State input; Derivatives output; I_ext input; excitatory_Vin input; inhibitory_Vin input; Params input
% This fcn implements the MQIF dynamics as ordinary differential equations.

function Derivatives = ODE(State, I_ext, excitatory_Vin, inhibitory_Vin, Params)
    % Parse through states
    V = State(1);
    Vs = State(2);
    Vus = State(3);
    Se = State(4:numel(excitatory_Vin)+3);
    Si = State(numel(excitatory_Vin)+4:end);

    % Parse through parameters
    g_f = Params(1);
    g_s = Params(2);
    g_us = Params(3);
    C = Params(4);
    tau_s = Params(5);
    tau_us = Params(6);
    tau_syn_E = Params(7);
    tau_syn_I = Params(8);
    Ve_syn = Params(9);
    Vi_syn = Params(10);
    g_syn_E = Params(11);
    g_syn_I = Params(12);
    Vin_gate_E = Params(13);
    Vin_gate_I = Params(14);
    k = Params(15);
    R = Params(16);
    V0 = Params(17);
    Vs0 = Params(18);
    Vus0 = Params(19);

    % Non-linear function to control synaptic gating
    sigmoid_Ve = 1./(1+exp(-(40*(excitatory_Vin-Vin_gate_E))));
    sigmoid_Vi = 1./(1+exp(-(40*(inhibitory_Vin-Vin_gate_I))));

    % Excitatory and inhibitory currents
    I_excitatory = g_syn_E*Se*(Ve_syn-V);
    I_inhibitory = g_syn_I*Si*(Vi_syn-V);

    % Passive Conductance in QuadCentre!!
    I_pass = (1/R)*(V-inhibitory_Vin(2));

    % ODE's that will be solved by the integrator block following this fcn
    V_dot = k*(((I_ext + g_f*((V-V0)^2) - g_s*((Vs-Vs0)^2) - g_us*((Vus-Vus0)^2) + sum(I_excitatory) + sum(I_inhibitory) + I_pass) / C));
    Vs_dot = k*((V - Vs) / tau_s);
    Vus_dot = k*((V - Vus) / tau_us);
    Se_dot = k*((sigmoid_Ve - Se)/tau_syn_E);
    Si_dot = k*((sigmoid_Vi - Si)/tau_syn_I);

    Derivatives = [V_dot; Vs_dot; Vus_dot; Se_dot; Si_dot];
end

== matlab function QuadCentreClosedCoupling/QuadCentre (Closed) CPG/HalfCentre CPG P/MQIF_Neuron A/MATLAB Function2 ==
  data: inputVector input; outputVector output
% This function is required to make sure that the MQIF neuron is input
% agnostic, (can handle any number of excitatory/inhibitory connections).
% 
% We require a matrix that can extract Vus (scalar), Se and Si (vectors of
% arbitrary length), and ignore the other values. This is because these
% values are "remembered" after each action potential and are required in
% the subsequent resetting of states.

function outputVector = generalisedMatrix(inputVector)
    % Get the size of the input vector
    n = length(inputVector);

    % Create a square matrix of zeros
    Matrix = zeros(n);

    % Set the (3, 3) element to 1
    Matrix(3, 3) = 1;

    % Set the values for every row i, starting from the fourth row
    for i = 4:n
        Matrix(i, i) = 1;
    end

    outputVector = Matrix*inputVector;
end

== matlab function QuadCentreClosedCoupling/QuadCentre (Closed) CPG/HalfCentre CPG P/MQIF_Neuron A/Parsing Function ==
  data: vector input; V output; Vs output; Vus output; Ve input; Se output; Si output
% This fcn parses through the vectorised input signal, to output the
% various states through the enclosing mask's outports. It is designed to
% be input agnostic, (i.e. the neuron can handle any number of excitatory/inhibitory
% connections, and it outputs Se and Si as vectorised signals).

function [V,Vs,Vus,Se,Si] = InputAgnosticDemux(vector, Ve)
    V = vector(1);
    Vs = vector(2);
    Vus = vector(3);
    Se = vector(4:numel(Ve)+3);
    Si = vector(numel(Ve)+4:end);
end

== matlab function QuadCentreClosedCoupling/QuadCentre (Closed) CPG/HalfCentre CPG Q/MQIF_Neuron A/MATLAB Function1 ==
  data: State input; Derivatives output; I_ext input; excitatory_Vin input; inhibitory_Vin input; Params input
% This fcn implements the MQIF dynamics as ordinary differential equations.

function Derivatives = ODE(State, I_ext, excitatory_Vin, inhibitory_Vin, Params)
    % Parse through states
    V = State(1);
    Vs = State(2);
    Vus = State(3);
    Se = State(4:numel(excitatory_Vin)+3);
    Si = State(numel(excitatory_Vin)+4:end);

    % Parse through parameters
    g_f = Params(1);
    g_s = Params(2);
    g_us = Params(3);
    C = Params(4);
    tau_s = Params(5);
    tau_us = Params(6);
    tau_syn_E = Params(7);
    tau_syn_I = Params(8);
    Ve_syn = Params(9);
    Vi_syn = Params(10);
    g_syn_E = Params(11);
    g_syn_I = Params(12);
    Vin_gate_E = Params(13);
    Vin_gate_I = Params(14);
    k = Params(15);
    R = Params(16);
    V0 = Params(17);
    Vs0 = Params(18);
    Vus0 = Params(19);

    % Non-linear function to control synaptic gating
    sigmoid_Ve = 1./(1+exp(-(40*(excitatory_Vin-Vin_gate_E))));
    sigmoid_Vi = 1./(1+exp(-(40*(inhibitory_Vin-Vin_gate_I))));

    % Excitatory and inhibitory currents
    I_excitatory = g_syn_E*Se*(Ve_syn-V);
    I_inhibitory = g_syn_I*Si*(Vi_syn-V);

    % Passive Conductance in QuadCentre!!
    I_pass = (1/R)*(V-inhibitory_Vin(2));

    % ODE's that will be solved by the integrator block following this fcn
    V_dot = k*(((I_ext + g_f*((V-V0)^2) - g_s*((Vs-Vs0)^2) - g_us*((Vus-Vus0)^2) + sum(I_excitatory) + sum(I_inhibitory) + I_pass) / C));
    Vs_dot = k*((V - Vs) / tau_s);
    Vus_dot = k*((V - Vus) / tau_us);
    Se_dot = k*((sigmoid_Ve - Se)/tau_syn_E);
    Si_dot = k*((sigmoid_Vi - Si)/tau_syn_I);

    Derivatives = [V_dot; Vs_dot; Vus_dot; Se_dot; Si_dot];
end

== matlab function QuadCentreClosedCoupling/QuadCentre (Closed) CPG/HalfCentre CPG Q/MQIF_Neuron A/MATLAB Function2 ==
  data: inputVector input; outputVector output
% This function is required to make sure that the MQIF neuron is input
% agnostic, (can handle any number of excitatory/inhibitory connections).
% 
% We require a matrix that can extract Vus (scalar), Se and Si (vectors of
% arbitrary length), and ignore the other values. This is because these
% values are "remembered" after each action potential and are required in
% the subsequent resetting of states.

function outputVector = generalisedMatrix(inputVector)
    % Get the size of the input vector
    n = length(inputVector);

    % Create a square matrix of zeros
    Matrix = zeros(n);

    % Set the (3, 3) element to 1
    Matrix(3, 3) = 1;

    % Set the values for every row i, starting from the fourth row
    for i = 4:n
        Matrix(i, i) = 1;
    end

    outputVector = Matrix*inputVector;
end

== matlab function QuadCentreClosedCoupling/QuadCentre (Closed) CPG/HalfCentre CPG Q/MQIF_Neuron A/Parsing Function ==
  data: vector input; V output; Vs output; Vus output; Ve input; Se output; Si output
% This fcn parses through the vectorised input signal, to output the
% various states through the enclosing mask's outports. It is designed to
% be input agnostic, (i.e. the neuron can handle any number of excitatory/inhibitory
% connections, and it outputs Se and Si as vectorised signals).

function [V,Vs,Vus,Se,Si] = InputAgnosticDemux(vector, Ve)
    V = vector(1);
    Vs = vector(2);
    Vus = vector(3);
    Se = vector(4:numel(Ve)+3);
    Si = vector(numel(Ve)+4:end);
end

== matlab function QuadCentreClosedCoupling/QuadCentre (Closed) CPG/HalfCentre CPG P/MQIF_Neuron B/MATLAB Function ==
  data: States input; reset output; V_threshold input
% This fcn triggers the reset of the following integrator block. When membrane
% potential rises above V_threshold, an action potential has been fired, 
% as specified for integrate-and-fire neuron behavior.

function reset = ResetTrigger(States, V_threshold)

V = States(1);

reset = (V > V_threshold);

end

== matlab function QuadCentreClosedCoupling/QuadCentre (Closed) CPG/HalfCentre CPG P/MQIF_Neuron B/MATLAB Function1 ==
  data: State input; Derivatives output; I_ext input; excitatory_Vin input; inhibitory_Vin input; Params input
% This fcn implements the MQIF dynamics as ordinary differential equations.

function Derivatives = ODE(State, I_ext, excitatory_Vin, inhibitory_Vin, Params)
    % Parse through states
    V = State(1);
    Vs = State(2);
    Vus = State(3);
    Se = State(4:numel(excitatory_Vin)+3);
    Si = State(numel(excitatory_Vin)+4:end);

    % Parse through parameters
    g_f = Params(1);
    g_s = Params(2);
    g_us = Params(3);
    C = Params(4);
    tau_s = Params(5);
    tau_us = Params(6);
    tau_syn_E = Params(7);
    tau_syn_I = Params(8);
    Ve_syn = Params(9);
    Vi_syn = Params(10);
    g_syn_E = Params(11);
    g_syn_I = Params(12);
    Vin_gate_E = Params(13);
    Vin_gate_I = Params(14);
    k = Params(15);
    R = Params(16);
    V0 = Params(17);
    Vs0 = Params(18);
    Vus0 = Params(19);

    % Non-linear function to control synaptic gating
    sigmoid_Ve = 1./(1+exp(-(40*(excitatory_Vin-Vin_gate_E))));
    sigmoid_Vi = 1./(1+exp(-(40*(inhibitory_Vin-Vin_gate_I))));

    % Excitatory and inhibitory currents
    I_excitatory = g_syn_E*Se*(Ve_syn-V);
    I_inhibitory = g_syn_I*Si*(Vi_syn-V);

    % Passive Conductance in QuadCentre!!
    I_pass = (1/R)*(V-inhibitory_Vin(2));

    % ODE's that will be solved by the integrator block following this fcn
    V_dot = k*(((I_ext + g_f*((V-V0)^2) - g_s*((Vs-Vs0)^2) - g_us*((Vus-Vus0)^2) + sum(I_excitatory) + sum(I_inhibitory) + I_pass) / C));
    Vs_dot = k*((V - Vs) / tau_s);
    Vus_dot = k*((V - Vus) / tau_us);
    Se_dot = k*((sigmoid_Ve - Se)/tau_syn_E);
    Si_dot = k*((sigmoid_Vi - Si)/tau_syn_I);

    Derivatives = [V_dot; Vs_dot; Vus_dot; Se_dot; Si_dot];
end

== matlab function QuadCentreClosedCoupling/QuadCentre (Closed) CPG/HalfCentre CPG P/MQIF_Neuron B/MATLAB Function2 ==
  data: inputVector input; outputVector output
% This function is required to make sure that the MQIF neuron is input
% agnostic, (can handle any number of excitatory/inhibitory connections).
% 
% We require a matrix that can extract Vus (scalar), Se and Si (vectors of
% arbitrary length), and ignore the other values. This is because these
% values are "remembered" after each action potential and are required in
% the subsequent resetting of states.

function outputVector = generalisedMatrix(inputVector)
    % Get the size of the input vector
    n = length(inputVector);

    % Create a square matrix of zeros
    Matrix = zeros(n);

    % Set the (3, 3) element to 1
    Matrix(3, 3) = 1;

    % Set the values for every row i, starting from the fourth row
    for i = 4:n
        Matrix(i, i) = 1;
    end

    outputVector = Matrix*inputVector;
end

== matlab function QuadCentreClosedCoupling/QuadCentre (Closed) CPG/HalfCentre CPG P/MQIF_Neuron B/Parsing Function ==
  data: vector input; V output; Vs output; Vus output; Ve input; Se output; Si output
% This fcn parses through the vectorised input signal, to output the
% various states through the enclosing mask's outports. It is designed to
% be input agnostic, (i.e. the neuron can handle any number of excitatory/inhibitory
% connections, and it outputs Se and Si as vectorised signals).

function [V,Vs,Vus,Se,Si] = InputAgnosticDemux(vector, Ve)
    V = vector(1);
    Vs = vector(2);
    Vus = vector(3);
    Se = vector(4:numel(Ve)+3);
    Si = vector(numel(Ve)+4:end);
end

== matlab function QuadCentreClosedCoupling/QuadCentre (Closed) CPG/HalfCentre CPG Q/MQIF_Neuron B/MATLAB Function ==
  data: States input; reset output; V_threshold input
% This fcn triggers the reset of the following integrator block. When membrane
% potential rises above V_threshold, an action potential has been fired, 
% as specified for integrate-and-fire neuron behavior.

function reset = ResetTrigger(States, V_threshold)

V = States(1);

reset = (V > V_threshold);

end

== matlab function QuadCentreClosedCoupling/QuadCentre (Closed) CPG/HalfCentre CPG Q/MQIF_Neuron B/MATLAB Function1 ==
  data: State input; Derivatives output; I_ext input; excitatory_Vin input; inhibitory_Vin input; Params input
% This fcn implements the MQIF dynamics as ordinary differential equations.

function Derivatives = ODE(State, I_ext, excitatory_Vin, inhibitory_Vin, Params)
    % Parse through states
    V = State(1);
    Vs = State(2);
    Vus = State(3);
    Se = State(4:numel(excitatory_Vin)+3);
    Si = State(numel(excitatory_Vin)+4:end);

    % Parse through parameters
    g_f = Params(1);
    g_s = Params(2);
    g_us = Params(3);
    C = Params(4);
    tau_s = Params(5);
    tau_us = Params(6);
    tau_syn_E = Params(7);
    tau_syn_I = Params(8);
    Ve_syn = Params(9);
    Vi_syn = Params(10);
    g_syn_E = Params(11);
    g_syn_I = Params(12);
    Vin_gate_E = Params(13);
    Vin_gate_I = Params(14);
    k = Params(15);
    R = Params(16);
    V0 = Params(17);
    Vs0 = Params(18);
    Vus0 = Params(19);

    % Non-linear function to control synaptic gating
    sigmoid_Ve = 1./(1+exp(-(40*(excitatory_Vin-Vin_gate_E))));
    sigmoid_Vi = 1./(1+exp(-(40*(inhibitory_Vin-Vin_gate_I))));

    % Excitatory and inhibitory currents
    I_excitatory = g_syn_E*Se*(Ve_syn-V);
    I_inhibitory = g_syn_I*Si*(Vi_syn-V);

    % Passive Conductance in QuadCentre!!
    I_pass = (1/R)*(V-inhibitory_Vin(2));

    % ODE's that will be solved by the integrator block following this fcn
    V_dot = k*(((I_ext + g_f*((V-V0)^2) - g_s*((Vs-Vs0)^2) - g_us*((Vus-Vus0)^2) + sum(I_excitatory) + sum(I_inhibitory) + I_pass) / C));
    Vs_dot = k*((V - Vs) / tau_s);
    Vus_dot = k*((V - Vus) / tau_us);
    Se_dot = k*((sigmoid_Ve - Se)/tau_syn_E);
    Si_dot = k*((sigmoid_Vi - Si)/tau_syn_I);

    Derivatives = [V_dot; Vs_dot; Vus_dot; Se_dot; Si_dot];
end
